simulink model "nonlinmodel"  (R2019b)
settings: Solver=VariableStepAuto  StartTime=0.0  StopTime=3000  RelTol=1e-3  EnableMultiTasking=on
values from neighbouring files (symbols this model uses):
  alpha = 0    [main.m]
  altitude = input('Enter the altitude for the simulation (ft)  :  ')    [main.m]
  Inertia = [9496,0,982 ... (first row only)    [main.m]
  mass = 636.94    [main.m]
  velocity = input('Enter the velocity for the simulation (ft/s):  ')    [main.m]
undefined symbols (not defined in the file or in its folder): U
libraries: aerolib6dof x4, simulink x4, aerolibobsolete x2, sharedutil x1
settings Model: Creator=Gray  LastModifiedBy=Administrator
settings DataIOCC: ReturnWorkspaceOutputs=off
settings OptimizationCC: LifeSpan=inf
settings DebuggingCC: SFUnexpectedBacktrackingDiag=warning  SFNoUnconditionalDefaultTransitionDiag=warning  ArithmeticOperatorsInVariantConditions=warning
settings SFSimCC: SimUseLocalCustomCode=off  CustomCodeUndefinedFunction=UseInterfaceOnly
settings RTWCC: RTWUseLocalCustomCode=off
settings CodeAppCC: StateflowObjectComments=on
settings GRTTargetCC: TargetLangStandard=C89/C90 (ANSI)  GeneratePreprocessorConditionals=Disable all
settings ConfigComp: CovMetricSettings=dw  CovHtmlReporting=on  CovSaveCumulativeToWorkspaceVar=on  CovSaveSingleToWorkspaceVar=on  CovExternalEMLEnable=off

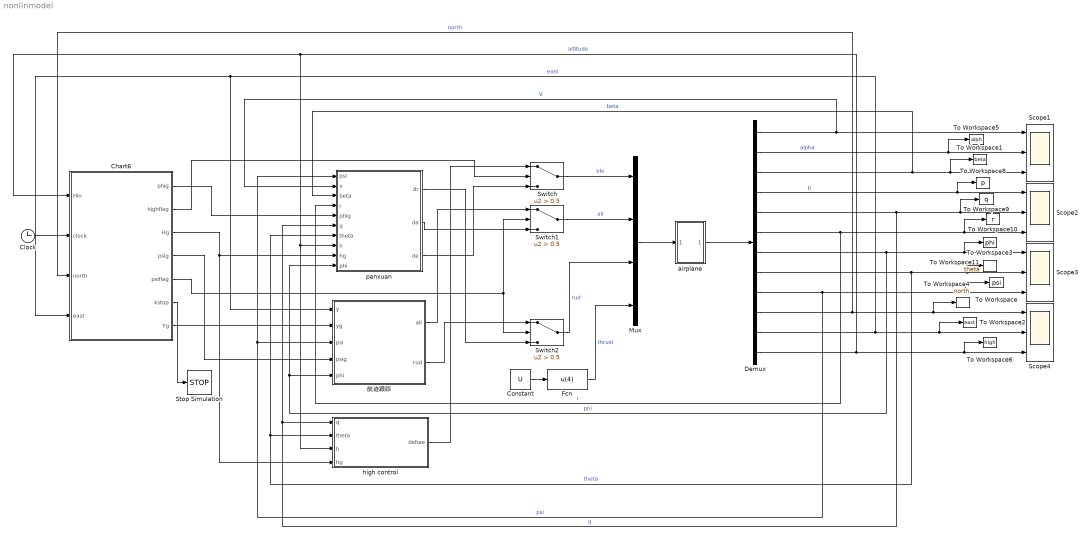
== system nonlinmodel ==
  Chart6 : Stateflow chart  TreatAsAtomicUnit=on
  Clock : Clock
  Constant : Constant  Value=U
  Demux : Demux  Outputs=12
  Fcn : Fcn  Expr=u(4)
  Mux : Mux
  Scope{1..4} (4 alike) : Scope  NumInputPorts=3
  Stop Simulation : Stop
  Switch : Switch  Criteria=u2 > Threshold  Threshold=0.5
  Switch1 : Switch  Criteria=u2 > Threshold  Threshold=0.5
  Switch2 : Switch  Criteria=u2 > Threshold  Threshold=0.5
  To Workspace : ToWorkspace  VariableName=psi  SaveFormat=Timeseries  SampleTime=-1
  To Workspace1 : ToWorkspace  VariableName=beta  SaveFormat=Timeseries  SampleTime=-1
  To Workspace10 : ToWorkspace  VariableName=r  SaveFormat=Timeseries  SampleTime=-1
  To Workspace11 : ToWorkspace  VariableName=theta  SaveFormat=Timeseries  SampleTime=-1
  To Workspace2 : ToWorkspace  VariableName=east  SampleTime=-1
  To Workspace3 : ToWorkspace  VariableName=phi  SaveFormat=Timeseries  SampleTime=-1
  To Workspace4 : ToWorkspace  VariableName=north  SampleTime=-1
  To Workspace5 : ToWorkspace  VariableName=alph  SaveFormat=Timeseries  SampleTime=-1
  To Workspace6 : ToWorkspace  VariableName=high  SampleTime=-1
      settings: Save2DSignal=2-D array (concatenate along first dimension)
  To Workspace8 : ToWorkspace  VariableName=p  SaveFormat=Timeseries  SampleTime=-1
  To Workspace9 : ToWorkspace  VariableName=q  SaveFormat=Timeseries  SampleTime=-1
  airplane : Subsystem
  high control : Subsystem
  panxuan : Subsystem
  航迹跟踪 : Subsystem
  wires:
  Demux/1 -> panxuan/2(v), Scope1/1  "V"
  Demux/2 -> To Workspace5/1, Scope1/2  "alpha"
  Demux/3 -> panxuan/3(beta), To Workspace1/1, Scope1/3  "beta"
  Demux/4 -> To Workspace8/1, Scope2/1  "p"
  Demux/5 -> panxuan/6(q), high control/1(q), To Workspace9/1, Scope2/2  "q"
  Demux/6 -> panxuan/4(r), To Workspace10/1, Scope2/3  "r"
  Demux/7 -> panxuan/10(phi), 航迹跟踪/5(phi), To Workspace3/1, Scope3/1  "phi"
  Demux/8 -> high control/2(theta), panxuan/7(theta), To Workspace11/1, Scope3/2  "theta"
  Demux/9 -> 航迹跟踪/3(psi), panxuan/1(psi), To Workspace/1, Scope3/3  "psi"
  Demux/10 -> Chart6/3(north), To Workspace4/1, Scope4/1  "north"
  Demux/11 -> Chart6/4(east), 航迹跟踪/1(y), To Workspace2/1, Scope4/2  "east"
  Demux/12 -> Chart6/1(Hin), high control/3(h), panxuan/8(h), To Workspace6/1, Scope4/3  "altitude"
  Fcn/1 -> Mux/4  "thrust"
  Chart6/1(phig) -> panxuan/5(phig)
  Chart6/3(Hg) -> high control/4(hg), panxuan/9(hg)
  Chart6/7(Yg) -> 航迹跟踪/2(yg)
  Chart6/4(psig) -> 航迹跟踪/4(psig)
  Switch/1 -> Mux/1  "ele"
  Switch1/1 -> Mux/2  "ail"
  Switch2/1 -> Mux/3  "rud"
  high control/1(deltae) -> Switch/1
  panxuan/3(de) -> Switch/3
  航迹跟踪/1(ail) -> Switch1/1
  panxuan/2(da) -> Switch1/3
  Chart6/2(highflag) -> Switch/2
  Chart6/5(psiflag) -> Switch2/2, Switch1/2
  Clock/1 -> Chart6/2(clock)
  Chart6/6(kstop) -> Stop Simulation/1
  航迹跟踪/2(rud) -> Switch2/1
  panxuan/1(dr) -> Switch2/3
  airplane/1(state) -> Demux/1
  Mux/1 -> airplane/1(In1)
  Constant/1 -> Fcn/1

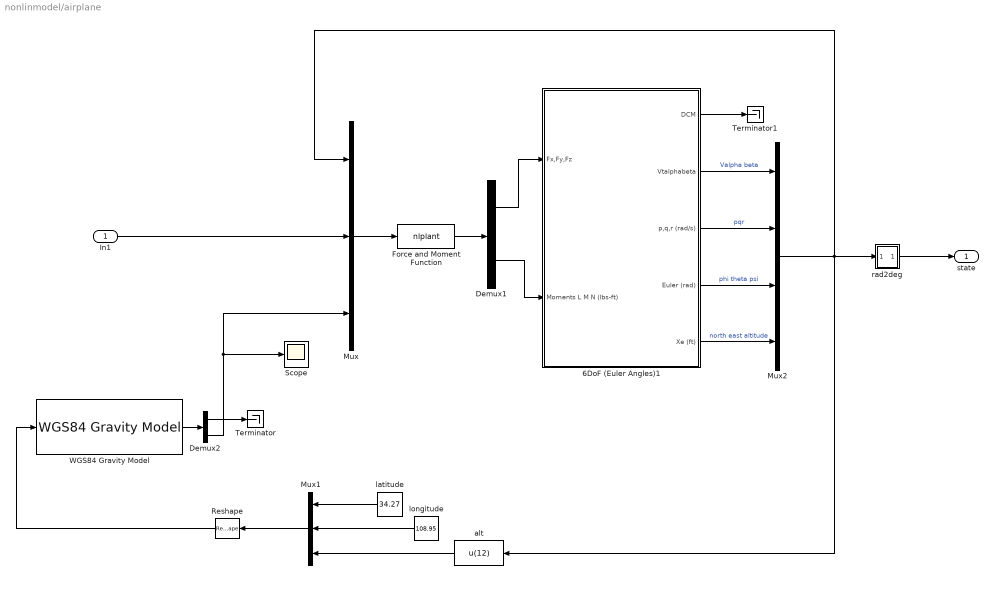
== system nonlinmodel/airplane ==
  In1 : Inport
  6DoF (Euler Angles)1 : Subsystem  RequirementInfo={} %GIDa_f78eee8a_25e5_4163_8dbf_11bc9aa697d0  AncestorBlock=aerolib6dof/6DoF (Euler Angles)  mask(6DoF (Euler Angles) EoM){xme_0=[0,0,altitude], Vmw_0=[velocity,alpha,0], eul_0=[0 0 0], pm_0=[0 0 0], mass=mass, Inertia=Inertia}
      mask prompts: xme_0 "Initial position in inertial axes [Xe,Ye,Ze] (ft):"; Vmw_0 "Vt  alpha  beta"; eul_0 "Initial Euler orientation [roll, pitch, yaw] (rad):"; pm_0 "Initial body rotation rates [p,q,r] (rad/s):"; mass "Mass (slugs):"; Inertia "Inertia matrix (slugs.ft^2):"
      mask help:
      | Integrate the six-degrees-of-freedom equations of motion using an Euler angle representation for the orientation of the body in space.
      |
      | Inputs are forces on the body in x-axis, y-axis, and z-axis; and moments on the body along x-axis, y-axis, and z-axis. Outputs are translational velocity in x-axis, y-axis, and z-axis in inertial coordinates; position in x-axis, y-axis, and z-axis in inertial coordinates; phi, theta, and psi; 3-by-3 direction cosine matrix; translational velocity in x-axis, y-axis, and z-axis in body coordinates; roll, pitch, and yaw rate; and roll, pitch, and yaw acceleration.
      mask Help: web(asbhelp('6dofeulerangles'));
      mask Display: disp('Euler\nAngles')
  Demux1 : Demux  Outputs=[3,3]
  Demux2 : Demux  Outputs=2
  Force and Moment Function : MATLABFcn  MATLABFcn=nlplant  OutputDimensions=6
  Mux : Mux  Inputs=[12,4,1]
  Mux1 : Mux  Inputs=3
  Mux2 : Mux
  Reshape : Reshape
  Scope : Scope
  Terminator : Terminator
  Terminator1 : Terminator
  "WGS84 Gravity Model " : aerolibobsolete/WGS84 Gravity Model   model=WGS84 Taylor Series  units=English  no_atmos=on  precessing=on  jd_loc=off  month=October  day=10  year=2004  no_centrifugal=on  action=Warning
      settings: SourceProductName=Aerospace Blockset  SourceProductBaseCode=AE
  alt : Fcn  Expr=u(12)
  latitude : Constant  Value=34.27
  longitude : Constant  Value=108.95
  rad2deg : Subsystem
  state : Outport
  wires:
  6DoF (Euler Angles)1/5(Xe (ft)) -> Mux2/4  "north east altitude"
  6DoF (Euler Angles)1/1(DCM) -> Terminator1/1
  rad2deg/1(Out1) -> state/1
  Force and Moment Function/1 -> Demux1/1
  latitude/1 -> Mux1/1
  Demux1/1 -> 6DoF (Euler Angles)1/1(Fx,Fy,Fz)
  Mux/1 -> Force and Moment Function/1
  In1/1 -> Mux/2
  Reshape/1 -> "WGS84 Gravity Model "/1
  alt/1 -> Mux1/3
  Demux1/2 -> 6DoF (Euler Angles)1/2(Moments L M N (lbs-ft))
  Demux2/2 -> Mux/3, Scope/1
  6DoF (Euler Angles)1/3(p,q,r (rad/s)) -> Mux2/2  "pqr"
  6DoF (Euler Angles)1/4(Euler (rad)) -> Mux2/3  "phi theta psi"
  Mux2/1 -> rad2deg/1(In1), alt/1, Mux/1
  longitude/1 -> Mux1/2
  Demux2/1 -> Terminator/1
  Mux1/1 -> Reshape/1
  "WGS84 Gravity Model "/1 -> Demux2/1
  6DoF (Euler Angles)1/2(Vtalphabeta) -> Mux2/1  "Valpha beta"

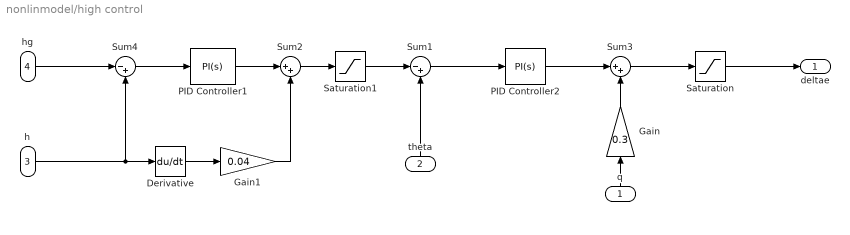
== system nonlinmodel/high control ==
  q : Inport
  theta : Inport  Port=2
  h : Inport  Port=3
  hg : Inport  Port=4
  Derivative : Derivative
  Gain : Gain  Gain=0.3
  Gain1 : Gain  Gain=0.04
  PID Controller1 : simulink/Continuous/PID Controller  Controller=PI  Form=Parallel  TimeDomain=Continuous-time  SampleTime=-1  IntegratorMethod=Forward Euler  FilterMethod=Forward Euler  ControllerParametersSource=internal  P=0.03  I=0.0002  D=0  UseFilter=on  N=100  TunerSelectOption=Transfer Function Based (PID Tuner App)  InitialConditionSource=internal  InitialConditionForIntegrator=0  InitialConditionForFilter=0  DifferentiatorICPrevScaledInput=0  ExternalReset=none  TrackingMode=off  Kt=1  LimitOutput=off  UpperSaturationLimit=inf  LowerSaturationLimit=-inf  LinearizeAsGain=on  AntiWindupMode=none  Kb=1  POutMin=[]  POutMax=[]  IOutMin=[]  IOutMax=[]  DOutMin=[]  DOutMax=[]  NOutMin=[]  NOutMax=[]  SumOutMin=[]  SumOutMax=[]  SaturationOutMin=[]  SaturationOutMax=[]  PParamMin=[]  PParamMax=[]  IParamMin=[]  IParamMax=[]  DParamMin=[]  DParamMax=[]  NParamMin=[]  NParamMax=[]  KbParamMin=[]  KbParamMax=[]  KtParamMin=[]  KtParamMax=[]  KbOutMin=[]  KbOutMax=[]  KtOutMin=[]  KtOutMax=[]  IntegratorOutMin=[]  IntegratorOutMax=[]  FilterOutMin=[]  FilterOutMax=[]  SumI1OutMin=[]  SumI1OutMax=[]  SumI2OutMin=[]  SumI2OutMax=[]  SumI3OutMin=[]  SumI3OutMax=[]  SumI4OutMin=[]  SumI4OutMax=[]  SumDOutMin=[]  SumDOutMax=[]  DifferentiatorOutMin=[]  DifferentiatorOutMax=[]  FilterDiffOutCoefMin=[]  FilterDiffOutCoefMax=[]  ReciprocalOutMin=[]  ReciprocalOutMax=[]  SumDenOutMin=[]  SumDenOutMax=[]  SumNumOutMin=[]  SumNumOutMax=[]  DivideOutMin=[]  DivideOutMax=[]  IntegratorContinuousStateAttributes=''  IntegratorStateMustResolveToSignalObject=off  IntegratorRTWStateStorageClass=Auto  FilterContinuousStateAttributes=''  FilterStateMustResolveToSignalObject=off  FilterRTWStateStorageClass=Auto  ParallelPVariant=InternalParameters  IdealPVariant=Disabled  IVariant=InternalParameters  DVariant=Disabled  IntegratorVariant=Continuous  SatVariant=Disabled  AWVariant=Passthrough  PCopyVariant=Disabled  TRVariant=Disabled  FdbkBlocksVariant=Forward  IdealPFdbkVariant=Disabled  SatFdbkVariant=Disabled  DerivativeFilterVariant=Disabled  NVariant=Disabled  NCopyVariant=Disabled_SignalSpec  FilterICVariant=Disabled  IntegratorICVariant=InternalICs  ExternalResetVariant=Disabled  TRSumVariant=Passthrough  SumFdbkVariant=Disabled  SumVariant=Sum_PI
  PID Controller2 : simulink/Continuous/PID Controller  Controller=PI  Form=Parallel  TimeDomain=Continuous-time  SampleTime=-1  IntegratorMethod=Forward Euler  FilterMethod=Forward Euler  ControllerParametersSource=internal  P=0.5  I=0  D=0  UseFilter=on  N=100  TunerSelectOption=Transfer Function Based (PID Tuner App)  InitialConditionSource=internal  InitialConditionForIntegrator=0  InitialConditionForFilter=0  DifferentiatorICPrevScaledInput=0  ExternalReset=none  TrackingMode=off  Kt=1  LimitOutput=off  UpperSaturationLimit=inf  LowerSaturationLimit=-inf  LinearizeAsGain=on  AntiWindupMode=none  Kb=1  POutMin=[]  POutMax=[]  IOutMin=[]  IOutMax=[]  DOutMin=[]  DOutMax=[]  NOutMin=[]  NOutMax=[]  SumOutMin=[]  SumOutMax=[]  SaturationOutMin=[]  SaturationOutMax=[]  PParamMin=[]  PParamMax=[]  IParamMin=[]  IParamMax=[]  DParamMin=[]  DParamMax=[]  NParamMin=[]  NParamMax=[]  KbParamMin=[]  KbParamMax=[]  KtParamMin=[]  KtParamMax=[]  KbOutMin=[]  KbOutMax=[]  KtOutMin=[]  KtOutMax=[]  IntegratorOutMin=[]  IntegratorOutMax=[]  FilterOutMin=[]  FilterOutMax=[]  SumI1OutMin=[]  SumI1OutMax=[]  SumI2OutMin=[]  SumI2OutMax=[]  SumI3OutMin=[]  SumI3OutMax=[]  SumI4OutMin=[]  SumI4OutMax=[]  SumDOutMin=[]  SumDOutMax=[]  DifferentiatorOutMin=[]  DifferentiatorOutMax=[]  FilterDiffOutCoefMin=[]  FilterDiffOutCoefMax=[]  ReciprocalOutMin=[]  ReciprocalOutMax=[]  SumDenOutMin=[]  SumDenOutMax=[]  SumNumOutMin=[]  SumNumOutMax=[]  DivideOutMin=[]  DivideOutMax=[]  IntegratorContinuousStateAttributes=''  IntegratorStateMustResolveToSignalObject=off  IntegratorRTWStateStorageClass=Auto  FilterContinuousStateAttributes=''  FilterStateMustResolveToSignalObject=off  FilterRTWStateStorageClass=Auto  ParallelPVariant=InternalParameters  IdealPVariant=Disabled  IVariant=InternalParameters  DVariant=Disabled  IntegratorVariant=Continuous  SatVariant=Disabled  AWVariant=Passthrough  PCopyVariant=Disabled  TRVariant=Disabled  FdbkBlocksVariant=Forward  IdealPFdbkVariant=Disabled  SatFdbkVariant=Disabled  DerivativeFilterVariant=Disabled  NVariant=Disabled  NCopyVariant=Disabled_SignalSpec  FilterICVariant=Disabled  IntegratorICVariant=InternalICs  ExternalResetVariant=Disabled  TRSumVariant=Passthrough  SumFdbkVariant=Disabled  SumVariant=Sum_PI
  Saturation : Saturate  UpperLimit=9  LowerLimit=-9
  Saturation1 : Saturate  UpperLimit=15  LowerLimit=-15
  Sum1 : Sum  Inputs=|-+
  Sum2 : Sum  Inputs=|++
  Sum3 : Sum  Inputs=|++
  Sum4 : Sum  Inputs=|-+
  deltae : Outport
  wires:
  hg/1 -> Sum4/1
  Sum4/1 -> PID Controller1/1
  PID Controller1/1 -> Sum2/1
  Sum1/1 -> PID Controller2/1
  PID Controller2/1 -> Sum3/1
  Sum3/1 -> Saturation/1
  h/1 -> Derivative/1, Sum4/2
  theta/1 -> Sum1/2
  Gain/1 -> Sum3/2
  q/1 -> Gain/1
  Saturation/1 -> deltae/1
  Saturation1/1 -> Sum1/1
  Sum2/1 -> Saturation1/1
  Derivative/1 -> Gain1/1
  Gain1/1 -> Sum2/2

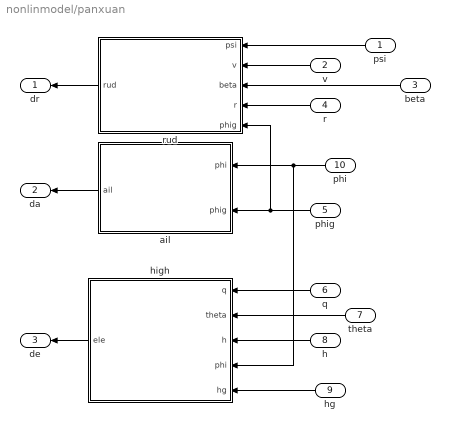
== system nonlinmodel/panxuan ==
  psi : Inport
  v : Inport  Port=2
  beta : Inport  Port=3
  r : Inport  Port=4
  phig : Inport  Port=5
  q : Inport  Port=6
  theta : Inport  Port=7
  h : Inport  Port=8
  hg : Inport  Port=9
  phi : Inport  Port=10
  ail : Subsystem
  "high " : Subsystem
  rud : Subsystem
  dr : Outport
  da : Outport  Port=2
  de : Outport  Port=3
  wires:
  psi/1 -> rud/1(psi)
  "high "/1(ele) -> de/1
  beta/1 -> rud/3(beta)
  r/1 -> rud/4(r)
  ail/1(ail) -> da/1
  v/1 -> rud/2(v)
  phig/1 -> rud/5(phig), ail/2(phig)
  theta/1 -> "high "/2(theta)
  q/1 -> "high "/1(q)
  h/1 -> "high "/3(h)
  hg/1 -> "high "/5(hg)
  rud/1(rud) -> dr/1
  phi/1 -> "high "/4(phi), ail/1(phi)

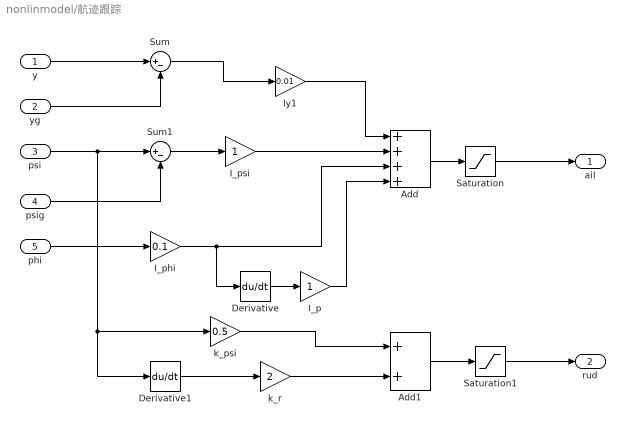
== system nonlinmodel/航迹跟踪 ==
  y : Inport
  yg : Inport  Port=2
  psi : Inport  Port=3
  psig : Inport  Port=4
  phi : Inport  Port=5
  Add : Sum  Inputs=++++
  Add1 : Sum
  Derivative : Derivative
  Derivative1 : Derivative
  I_p : Gain
  I_phi : Gain  Gain=0.1
  I_psi : Gain
  Iy1 : Gain  Gain=0.01
  Saturation : Saturate  UpperLimit=12  LowerLimit=-12
  Saturation1 : Saturate  UpperLimit=8  LowerLimit=-8
  Sum : Sum  Inputs=|+-
  Sum1 : Sum  Inputs=|+-
  k_psi : Gain  Gain=0.5
  k_r : Gain  Gain=2
  ail : Outport
  rud : Outport  Port=2
  wires:
  k_r/1 -> Add1/2
  k_psi/1 -> Add1/1
  Sum1/1 -> I_psi/1
  Add/1 -> Saturation/1
  Saturation/1 -> ail/1
  Add1/1 -> Saturation1/1
  Sum/1 -> Iy1/1
  Iy1/1 -> Add/1
  psi/1 -> Derivative1/1, k_psi/1, Sum1/1
  y/1 -> Sum/1
  psig/1 -> Sum1/2
  phi/1 -> I_phi/1
  I_phi/1 -> Derivative/1, Add/3
  Derivative/1 -> I_p/1
  Derivative1/1 -> k_r/1
  Saturation1/1 -> rud/1
  I_psi/1 -> Add/2
  I_p/1 -> Add/4
  yg/1 -> Sum/2

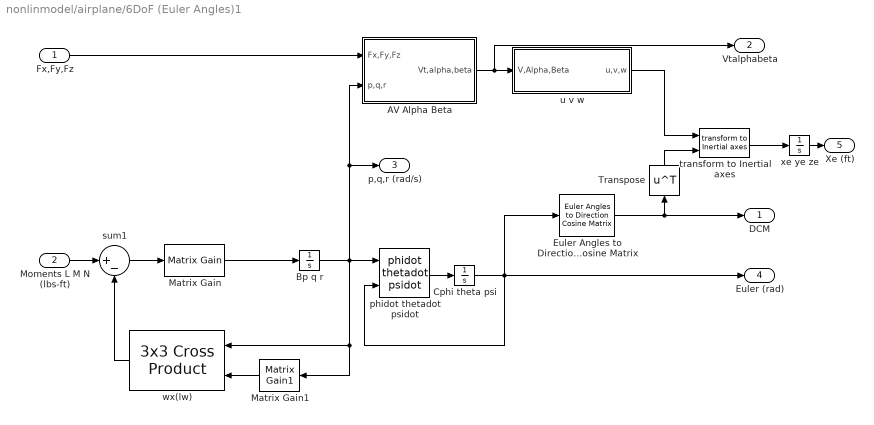
== system nonlinmodel/airplane/6DoF (Euler Angles)1 ==
  Fx,Fy,Fz : Inport  RequirementInfo={} %GIDa_47575797_6420_4b0e_a3a2_58bd686c73d1
  Moments L M N (lbs-ft) : Inport  RequirementInfo={} %GIDa_a1310ba6_e4bb_4a22_a342_2a9731745c55  Port=2
  AV Alpha Beta : Subsystem  RequirementInfo={} %GIDa_3bec4ccc_780c_4f29_8155_577fd785963f
  Bp q r : Integrator  RequirementInfo={} %GIDa_acd68407_7d65_4437_a75f_12a6524d518c  InitialCondition=pm_0
  Cphi theta psi : Integrator  RequirementInfo={} %GIDa_14df3cec_9b2c_44ff_9ee3_5db495ed21e4  InitialCondition=eul_0
  Euler Angles to Direction Cosine Matrix : aerolibobsolete/Euler Angles to  Direction Cosine Matrix
      settings: SourceProductName=Aerospace Blockset  SourceProductBaseCode=AE
  Matrix Gain : aerolib6dof/6DoF (Euler Angles)/Matrix Gain  K=inv(Inertia)
      settings: SourceProductName=Aerospace Blockset  SourceProductBaseCode=AE
  Matrix Gain1 : aerolib6dof/6DoF (Euler Angles)/Matrix Gain1  K=Inertia
      settings: SourceProductName=Aerospace Blockset  SourceProductBaseCode=AE
  Transpose : Math  RequirementInfo={} %GIDa_05e2ce72_03a0_43ff_82ff_9bf5926046c8  Operator=transpose  SaturateOnIntegerOverflow=on
  phidot thetadot psidot : aerolib6dof/6DoF (Euler Angles)/phidot thetadot psidot  SystemSampleTime=-1  Latency=0  AutoFrameSizeCalculation=off
      settings: SourceProductName=Aerospace Blockset  SourceProductBaseCode=AE
  sum1 : Sum  RequirementInfo={} %GIDa_32be784a_f452_4b23_b55c_981dfbd798a6  Inputs=|+-  SaturateOnIntegerOverflow=on  InputSameDT=on  OutDataTypeStr=Inherit: Same as first input
  "transform to Inertial axes " : aerolib6dof/6DoF (Euler Angles)/transform to Inertial axes   SystemSampleTime=-1  Latency=0  AutoFrameSizeCalculation=off
      settings: SourceProductName=Aerospace Blockset  SourceProductBaseCode=AE
  u v w : Subsystem  RequirementInfo={} %GIDa_bf3c1f97_35ea_453e_a36d_366a8121257e
  wx(lw) : sharedutil/3x3 Cross Product  aMode=aMode
      settings: SourceProductBaseCode=AE
  xe ye ze : Integrator  RequirementInfo={} %GIDa_cfcfa943_adf2_4818_a2ff_e6c6db1ce85e  InitialCondition=xme_0
  DCM : Outport  RequirementInfo={} %GIDa_e636d6ae_e403_4b09_a804_1aa986cdae3b
  Vtalphabeta : Outport  RequirementInfo={} %GIDa_aa55a071_a531_47c1_a623_ce86d5a78c20  Port=2
  p,q,r (rad/s) : Outport  RequirementInfo={} %GIDa_fd949a73_e74c_4d0d_912e_86edec8a02c0  Port=3
  Euler (rad) : Outport  RequirementInfo={} %GIDa_0d674778_96dd_4688_9946_da01fc5c90ef  Port=4
  Xe (ft) : Outport  RequirementInfo={} %GIDa_d3340636_7588_4a71_8e89_73856e7a4ca7  Port=5
  wires:
  Transpose/1 -> "transform to Inertial axes "/2
  Euler Angles to Direction Cosine Matrix/1 -> Transpose/1, DCM/1
  Matrix Gain/1 -> Bp q r/1
  wx(lw)/1 -> sum1/2
  Matrix Gain1/1 -> wx(lw)/2
  Moments L M N (lbs-ft)/1 -> sum1/1
  sum1/1 -> Matrix Gain/1
  Bp q r/1 -> Matrix Gain1/1, wx(lw)/1, phidot thetadot psidot/1, p,q,r (rad/s)/1, AV Alpha Beta/2(p,q,r)
  "transform to Inertial axes "/1 -> xe ye ze/1
  xe ye ze/1 -> Xe (ft)/1
  u v w/1(u,v,w) -> "transform to Inertial axes "/1
  Cphi theta psi/1 -> phidot thetadot psidot/2, Euler Angles to Direction Cosine Matrix/1, Euler (rad)/1
  phidot thetadot psidot/1 -> Cphi theta psi/1
  AV Alpha Beta/1(Vt,alpha,beta) -> Vtalphabeta/1, u v w/1(V,Alpha,Beta)
  Fx,Fy,Fz/1 -> AV Alpha Beta/1(Fx,Fy,Fz)

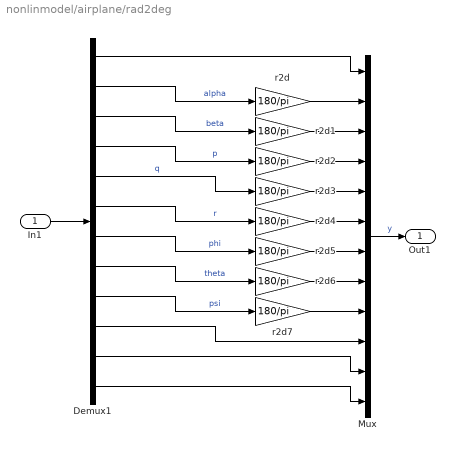
== system nonlinmodel/airplane/rad2deg ==
  In1 : Inport
  Demux1 : Demux  Outputs=12
  Mux : Mux  Inputs=12
  r2d{,1..7} (8 alike) : Gain  Gain=180/pi  SaturateOnIntegerOverflow=on  OutDataTypeStr=Inherit: Same as input  ParamDataTypeStr=Inherit: Same as input
  Out1 : Outport
  wires:
  In1/1 -> Demux1/1
  r2d2/1 -> Mux/4
  r2d1/1 -> Mux/3
  r2d/1 -> Mux/2
  Mux/1 -> Out1/1  "y"
  Demux1/1 -> Mux/1
  Demux1/2 -> r2d/1  "alpha"
  Demux1/3 -> r2d1/1  "beta"
  Demux1/4 -> r2d2/1  "p"
  Demux1/5 -> r2d3/1  "q"
  r2d3/1 -> Mux/5
  r2d4/1 -> Mux/6
  r2d5/1 -> Mux/7
  r2d6/1 -> Mux/8
  r2d7/1 -> Mux/9
  Demux1/6 -> r2d4/1  "r"
  Demux1/7 -> r2d5/1  "phi"
  Demux1/8 -> r2d6/1  "theta"
  Demux1/9 -> r2d7/1  "psi"
  Demux1/10 -> Mux/10
  Demux1/11 -> Mux/11
  Demux1/12 -> Mux/12

== system nonlinmodel/panxuan/ail ==
  phi : Inport
  phig : Inport  Port=2
  Add : Sum  Inputs=-+
  Add1 : Sum  Inputs=+++
  Derivative : Derivative
  Gain1 : Gain  Gain=0.4
  Gain2 : Gain
  Gain3 : Gain
  Integrator : Integrator
  Saturation : Saturate  UpperLimit=12  LowerLimit=-12
  ail : Outport
  wires:
  phi/1 -> Derivative/1, Add/2, Gain2/1
  Add1/1 -> Saturation/1
  Add/1 -> Integrator/1
  Integrator/1 -> Gain1/1
  Saturation/1 -> ail/1
  phig/1 -> Add/1
  Derivative/1 -> Gain3/1
  Gain2/1 -> Add1/2
  Gain3/1 -> Add1/3
  Gain1/1 -> Add1/1

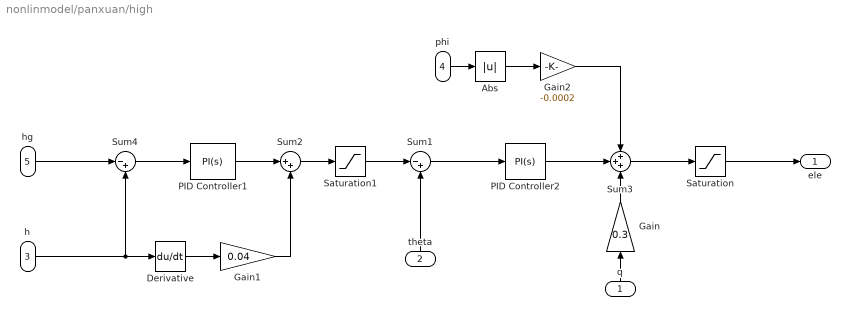
== system nonlinmodel/panxuan/high  ==
  q : Inport
  theta : Inport  Port=2
  h : Inport  Port=3
  phi : Inport  Port=4
  hg : Inport  Port=5
  Abs : Abs
  Derivative : Derivative
  Gain : Gain  Gain=0.3
  Gain1 : Gain  Gain=0.04
  Gain2 : Gain  Gain=-0.0002
  PID Controller1 : simulink/Continuous/PID Controller  Controller=PI  Form=Parallel  TimeDomain=Continuous-time  SampleTime=-1  IntegratorMethod=Forward Euler  FilterMethod=Forward Euler  ControllerParametersSource=internal  P=0.03  I=0.0002  D=0  UseFilter=on  N=100  TunerSelectOption=Transfer Function Based (PID Tuner App)  InitialConditionSource=internal  InitialConditionForIntegrator=0  InitialConditionForFilter=0  DifferentiatorICPrevScaledInput=0  ExternalReset=none  TrackingMode=off  Kt=1  LimitOutput=off  UpperSaturationLimit=inf  LowerSaturationLimit=-inf  LinearizeAsGain=on  AntiWindupMode=none  Kb=1  POutMin=[]  POutMax=[]  IOutMin=[]  IOutMax=[]  DOutMin=[]  DOutMax=[]  NOutMin=[]  NOutMax=[]  SumOutMin=[]  SumOutMax=[]  SaturationOutMin=[]  SaturationOutMax=[]  PParamMin=[]  PParamMax=[]  IParamMin=[]  IParamMax=[]  DParamMin=[]  DParamMax=[]  NParamMin=[]  NParamMax=[]  KbParamMin=[]  KbParamMax=[]  KtParamMin=[]  KtParamMax=[]  KbOutMin=[]  KbOutMax=[]  KtOutMin=[]  KtOutMax=[]  IntegratorOutMin=[]  IntegratorOutMax=[]  FilterOutMin=[]  FilterOutMax=[]  SumI1OutMin=[]  SumI1OutMax=[]  SumI2OutMin=[]  SumI2OutMax=[]  SumI3OutMin=[]  SumI3OutMax=[]  SumI4OutMin=[]  SumI4OutMax=[]  SumDOutMin=[]  SumDOutMax=[]  DifferentiatorOutMin=[]  DifferentiatorOutMax=[]  FilterDiffOutCoefMin=[]  FilterDiffOutCoefMax=[]  ReciprocalOutMin=[]  ReciprocalOutMax=[]  SumDenOutMin=[]  SumDenOutMax=[]  SumNumOutMin=[]  SumNumOutMax=[]  DivideOutMin=[]  DivideOutMax=[]  IntegratorContinuousStateAttributes=''  IntegratorStateMustResolveToSignalObject=off  IntegratorRTWStateStorageClass=Auto  FilterContinuousStateAttributes=''  FilterStateMustResolveToSignalObject=off  FilterRTWStateStorageClass=Auto  ParallelPVariant=InternalParameters  IdealPVariant=Disabled  IVariant=InternalParameters  DVariant=Disabled  IntegratorVariant=Continuous  SatVariant=Disabled  AWVariant=Passthrough  PCopyVariant=Disabled  TRVariant=Disabled  FdbkBlocksVariant=Forward  IdealPFdbkVariant=Disabled  SatFdbkVariant=Disabled  DerivativeFilterVariant=Disabled  NVariant=Disabled  NCopyVariant=Disabled_SignalSpec  FilterICVariant=Disabled  IntegratorICVariant=InternalICs  ExternalResetVariant=Disabled  TRSumVariant=Passthrough  SumFdbkVariant=Disabled  SumVariant=Sum_PI
  PID Controller2 : simulink/Continuous/PID Controller  Controller=PI  Form=Parallel  TimeDomain=Continuous-time  SampleTime=-1  IntegratorMethod=Forward Euler  FilterMethod=Forward Euler  ControllerParametersSource=internal  P=0.5  I=0  D=0  UseFilter=on  N=100  TunerSelectOption=Transfer Function Based (PID Tuner App)  InitialConditionSource=internal  InitialConditionForIntegrator=0  InitialConditionForFilter=0  DifferentiatorICPrevScaledInput=0  ExternalReset=none  TrackingMode=off  Kt=1  LimitOutput=off  UpperSaturationLimit=inf  LowerSaturationLimit=-inf  LinearizeAsGain=on  AntiWindupMode=none  Kb=1  POutMin=[]  POutMax=[]  IOutMin=[]  IOutMax=[]  DOutMin=[]  DOutMax=[]  NOutMin=[]  NOutMax=[]  SumOutMin=[]  SumOutMax=[]  SaturationOutMin=[]  SaturationOutMax=[]  PParamMin=[]  PParamMax=[]  IParamMin=[]  IParamMax=[]  DParamMin=[]  DParamMax=[]  NParamMin=[]  NParamMax=[]  KbParamMin=[]  KbParamMax=[]  KtParamMin=[]  KtParamMax=[]  KbOutMin=[]  KbOutMax=[]  KtOutMin=[]  KtOutMax=[]  IntegratorOutMin=[]  IntegratorOutMax=[]  FilterOutMin=[]  FilterOutMax=[]  SumI1OutMin=[]  SumI1OutMax=[]  SumI2OutMin=[]  SumI2OutMax=[]  SumI3OutMin=[]  SumI3OutMax=[]  SumI4OutMin=[]  SumI4OutMax=[]  SumDOutMin=[]  SumDOutMax=[]  DifferentiatorOutMin=[]  DifferentiatorOutMax=[]  FilterDiffOutCoefMin=[]  FilterDiffOutCoefMax=[]  ReciprocalOutMin=[]  ReciprocalOutMax=[]  SumDenOutMin=[]  SumDenOutMax=[]  SumNumOutMin=[]  SumNumOutMax=[]  DivideOutMin=[]  DivideOutMax=[]  IntegratorContinuousStateAttributes=''  IntegratorStateMustResolveToSignalObject=off  IntegratorRTWStateStorageClass=Auto  FilterContinuousStateAttributes=''  FilterStateMustResolveToSignalObject=off  FilterRTWStateStorageClass=Auto  ParallelPVariant=InternalParameters  IdealPVariant=Disabled  IVariant=InternalParameters  DVariant=Disabled  IntegratorVariant=Continuous  SatVariant=Disabled  AWVariant=Passthrough  PCopyVariant=Disabled  TRVariant=Disabled  FdbkBlocksVariant=Forward  IdealPFdbkVariant=Disabled  SatFdbkVariant=Disabled  DerivativeFilterVariant=Disabled  NVariant=Disabled  NCopyVariant=Disabled_SignalSpec  FilterICVariant=Disabled  IntegratorICVariant=InternalICs  ExternalResetVariant=Disabled  TRSumVariant=Passthrough  SumFdbkVariant=Disabled  SumVariant=Sum_PI
  Saturation : Saturate  UpperLimit=9  LowerLimit=-9
  Saturation1 : Saturate  UpperLimit=15  LowerLimit=-15
  Sum1 : Sum  Inputs=|-+
  Sum2 : Sum  Inputs=|++
  Sum3 : Sum  Inputs=+++
  Sum4 : Sum  Inputs=|-+
  ele : Outport
  wires:
  hg/1 -> Sum4/1
  Sum4/1 -> PID Controller1/1
  PID Controller1/1 -> Sum2/1
  Sum1/1 -> PID Controller2/1
  Sum3/1 -> Saturation/1
  h/1 -> Derivative/1, Sum4/2
  theta/1 -> Sum1/2
  q/1 -> Gain/1
  Saturation/1 -> ele/1
  Saturation1/1 -> Sum1/1
  Sum2/1 -> Saturation1/1
  Derivative/1 -> Gain1/1
  Gain1/1 -> Sum2/2
  PID Controller2/1 -> Sum3/2
  Gain/1 -> Sum3/3
  phi/1 -> Abs/1
  Abs/1 -> Gain2/1
  Gain2/1 -> Sum3/1

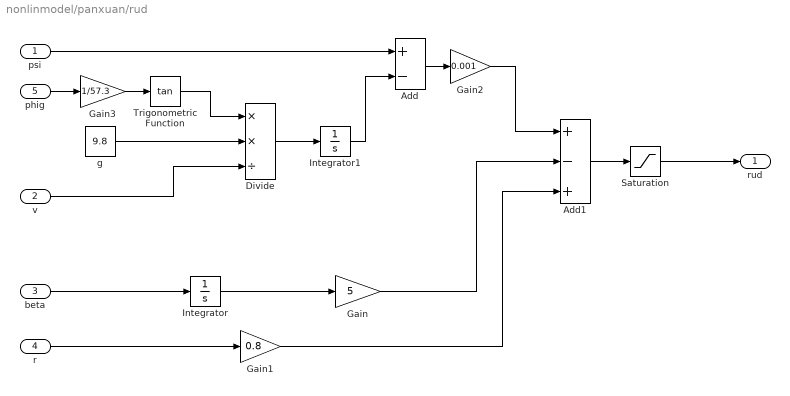
== system nonlinmodel/panxuan/rud ==
  psi : Inport
  v : Inport  Port=2
  beta : Inport  Port=3
  r : Inport  Port=4
  phig : Inport  Port=5
  Add : Sum  Inputs=+-
  Add1 : Sum  Inputs=+-+
  Divide : Product  Inputs=**/
  Gain : Gain  Gain=5
  Gain1 : Gain  Gain=0.8
  Gain2 : Gain  Gain=0.001
  Gain3 : Gain  Gain=1/57.3
  Integrator : Integrator
  Integrator1 : Integrator
  Saturation : Saturate  UpperLimit=8  LowerLimit=-8
  Trigonometric Function : Trigonometry  Operator=tan
  g : Constant  Value=9.8
  rud : Outport
  wires:
  Saturation/1 -> rud/1
  Add1/1 -> Saturation/1
  Trigonometric Function/1 -> Divide/1
  g/1 -> Divide/2
  psi/1 -> Add/1
  Add/1 -> Gain2/1
  r/1 -> Gain1/1
  Divide/1 -> Integrator1/1
  Integrator1/1 -> Add/2
  v/1 -> Divide/3
  Gain1/1 -> Add1/3
  Integrator/1 -> Gain/1
  beta/1 -> Integrator/1
  Gain2/1 -> Add1/1
  Gain/1 -> Add1/2
  phig/1 -> Gain3/1
  Gain3/1 -> Trigonometric Function/1

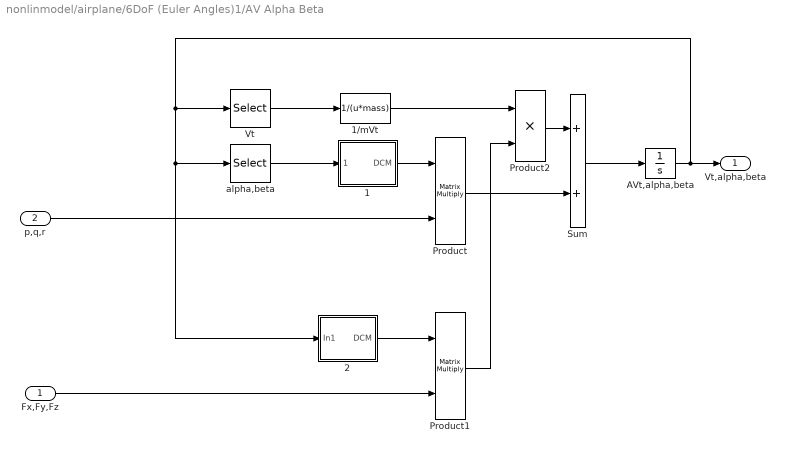
== system nonlinmodel/airplane/6DoF (Euler Angles)1/AV Alpha Beta ==
  Fx,Fy,Fz : Inport  RequirementInfo={} %GIDa_3a0cf2a3_c1ed_4a73_94fd_889fed1d9b56
  p,q,r : Inport  RequirementInfo={} %GIDa_a5f9e550_3eab_4ac3_94b5_06fdd9a422da  Port=2
  1 : Subsystem  RequirementInfo={} %GIDa_c99e5cc3_cc96_42d4_9ef2_1efd010a1b78  AncestorBlock="aerolibtransform/Euler Angles to  Direction Cosine Matrix"  mask(Euler2DCM){}
      mask help: Determine the 3-by-3 direction cosine matrix (DCM) from an Euler orientation (roll, pitch, yaw). The output DCM transforms vectors from inertial axes to body axes.
      mask Help: web(asbhelp('euleranglestodirectioncosinematrix'));
      mask Display: disp('Eul2DCM')
  1/mVt : Fcn  RequirementInfo={} %GIDa_624a88a3_87d0_4b9d_baa6_8a4cfcde3bec  Expr=1/(u*mass)
  2 : Subsystem  RequirementInfo={} %GIDa_e3eb13bd_00a3_4e12_afed_b34375ccdab9  AncestorBlock="aerolibtransform/Euler Angles to  Direction Cosine Matrix"  mask(Euler2DCM){}
      mask help: Determine the 3-by-3 direction cosine matrix (DCM) from an Euler orientation (roll, pitch, yaw). The output DCM transforms vectors from inertial axes to body axes.
      mask Help: web(asbhelp('euleranglestodirectioncosinematrix'));
      mask Display: disp('Eul2DCM')
  AVt,alpha,beta : Integrator  RequirementInfo={} %GIDa_5872e78a_3bc5_4f03_9b8b_91f33d6f31ba  InitialCondition=Vmw_0
  Product : Product  RequirementInfo={} %GIDa_2274bb0d_f78c_488a_822a_45d167d88f93  Multiplication=Matrix(*)  SaturateOnIntegerOverflow=on  OutDataTypeStr=Inherit: Same as first input
  Product1 : Product  RequirementInfo={} %GIDa_0f8d436f_1e01_4328_91a6_d2bc540051ee  Multiplication=Matrix(*)  SaturateOnIntegerOverflow=on  OutDataTypeStr=Inherit: Same as first input
  Product2 : Product  RequirementInfo={} %GIDa_e5f757ea_6d25_4229_bd39_4205d2ac714e  SaturateOnIntegerOverflow=on  OutDataTypeStr=Inherit: Same as first input
  Sum : Sum  RequirementInfo={} %GIDa_dca47486_89f6_482a_88b1_b8e711c95790  SaturateOnIntegerOverflow=on
  Vt : Selector  RequirementInfo={} %GIDa_5895aaee_ce00_487e_a691_99d90d7f70b9  InputPortWidth=3  IndexOptions=Index vector (dialog)  Indices=[1]  OutputSizes=1
  alpha,beta : Selector  RequirementInfo={} %GIDa_af6a7055_0671_43e6_ae58_ce8d0b3d3dfc  InputPortWidth=3  IndexOptions=Index vector (dialog)  Indices=[2 3]  OutputSizes=1
  Vt,alpha,beta : Outport  RequirementInfo={} %GIDa_cdaa0784_0bf0_4f30_8d27_66f252016894
  wires:
  1/1(DCM) -> Product/1
  p,q,r/1 -> Product/2
  2/1(DCM) -> Product1/1
  alpha,beta/1 -> 1/1(aeodata)
  Fx,Fy,Fz/1 -> Product1/2
  Vt/1 -> 1/mVt/1
  Product1/1 -> Product2/2
  1/mVt/1 -> Product2/1
  Product2/1 -> Sum/1
  Product/1 -> Sum/2
  Sum/1 -> AVt,alpha,beta/1
  AVt,alpha,beta/1 -> Vt,alpha,beta/1, Vt/1, 2/1(In1), alpha,beta/1

== system nonlinmodel/airplane/6DoF (Euler Angles)1/u v w ==
  V,Alpha,Beta : Inport  RequirementInfo={} %GIDa_c914807c_377c_4805_904c_b9dd6b416fbe
  11 : Fcn  RequirementInfo={} %GIDa_d585e0af_bb62_4f73_bfd9_c6723cca6caa  Expr=u(3)*u(4)*u(5)
  21 : Fcn  RequirementInfo={} %GIDa_43b00716_1676_4525_a1fa_24f1ca32aa06  Expr=u(2)*u(5)
  31 : Fcn  RequirementInfo={} %GIDa_18e180b3_585b_4d34_a8cd_b377e391badc  Expr=u(1)*u(4)*u(5)
  Demux : Demux  RequirementInfo={} %GIDa_6872fdb6_9740_423d_ad70_4060b7917c22  Outputs=[1,2]
  Mux : Mux  RequirementInfo={} %GIDa_6855cb8d_5fe5_474e_adbb_e3179ac4eebe  Inputs=3
  Mux1 : Mux  RequirementInfo={} %GIDa_6d5c0bc9_39df_4fb1_b18d_a12a1f469acd  Inputs=3
  cos(alpha,beta) : Trigonometry  RequirementInfo={} %GIDa_de370d12_4345_49dc_94a0_85fda68f9318  Operator=cos
  sin(alpha,beta) : Trigonometry  RequirementInfo={} %GIDa_6f775f89_370c_4c24_bd51_5746d9ad32c3
  u,v,w : Outport  RequirementInfo={} %GIDa_faedc8a5_0e93_4459_a6c9_fe783164ef2e
  wires:
  V,Alpha,Beta/1 -> Demux/1
  Mux1/1 -> u,v,w/1
  sin(alpha,beta)/1 -> Mux/1
  cos(alpha,beta)/1 -> Mux/2
  Mux/1 -> 11/1, 21/1, 31/1
  Demux/1 -> Mux/3
  11/1 -> Mux1/1
  21/1 -> Mux1/2
  31/1 -> Mux1/3
  Demux/2 -> sin(alpha,beta)/1, cos(alpha,beta)/1

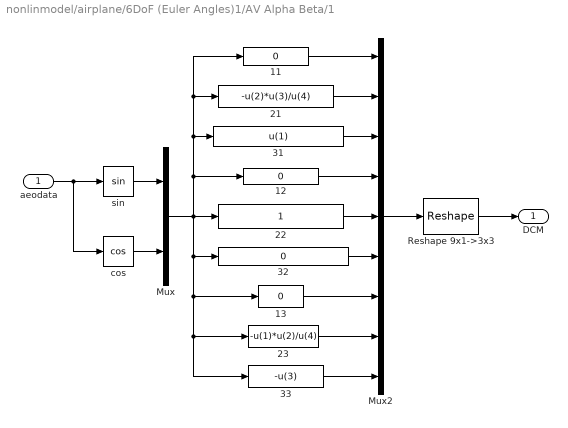
== system nonlinmodel/airplane/6DoF (Euler Angles)1/AV Alpha Beta/1 ==
  aeodata : Inport  RequirementInfo={} %GIDa_26334d88_e482_484f_b2e7_c9fa6d526c27
  11 : Fcn  RequirementInfo={} %GIDa_3b64c8f2_ebc0_426a_a0b0_8d1b09163b48  Expr=0
  12 : Fcn  RequirementInfo={} %GIDa_62435e47_a87c_4dcd_b50e_177845bffaf0  Expr=0
  13 : Fcn  RequirementInfo={} %GIDa_1b5cde54_80f2_453f_8970_fe6aea009974  Expr=0
  21 : Fcn  RequirementInfo={} %GIDa_bd0fbc7c_0fa4_407c_a960_55cbadc205e2  Expr=-u(2)*u(3)/u(4)
  22 : Fcn  RequirementInfo={} %GIDa_b9d67027_81e2_441a_be1e_54c25a531490  Expr=1
  23 : Fcn  RequirementInfo={} %GIDa_5b34ddd2_f10b_46f3_a37d_d3db88c149ce  Expr=-u(1)*u(2)/u(4)
  31 : Fcn  RequirementInfo={} %GIDa_c0edd0fb_54b7_4d9b_996f_cd482e49dd82  Expr=u(1)
  32 : Fcn  RequirementInfo={} %GIDa_f063a6a6_3071_4678_ae87_0d85f85bf8e7  Expr=0
  33 : Fcn  RequirementInfo={} %GIDa_8e91e91c_cea0_4225_b517_e6ef505d02c9  Expr=-u(3)
  Mux : Mux  RequirementInfo={} %GIDa_533c009e_0b36_44d6_89a0_d85a9332b8c0  Inputs=2
  Mux2 : Mux  RequirementInfo={} %GIDa_01f06579_276f_4188_a891_ef4ef8fa48ef  Inputs=9
  Reshape 9x1->3x3 : Reshape  RequirementInfo={} %GIDa_f87fc956_d370_46d1_9810_e7adad4a2eed  OutputDimensionality=Customize  OutputDimensions=[3,3]
  cos : Trigonometry  RequirementInfo={} %GIDa_e724210f_fb03_4dde_aece_76312382e649  Operator=cos
  sin : Trigonometry  RequirementInfo={} %GIDa_e4915e86_d752_4f6e_aa35_24073a1246c8
  DCM : Outport  RequirementInfo={} %GIDa_0ccdfa7e_6a60_431c_9fd0_97638da1abe3  InitialOutput=0
  wires:
  33/1 -> Mux2/9
  23/1 -> Mux2/8
  13/1 -> Mux2/7
  32/1 -> Mux2/6
  22/1 -> Mux2/5
  12/1 -> Mux2/4
  31/1 -> Mux2/3
  21/1 -> Mux2/2
  11/1 -> Mux2/1
  Mux2/1 -> Reshape 9x1->3x3/1
  Reshape 9x1->3x3/1 -> DCM/1
  sin/1 -> Mux/1
  cos/1 -> Mux/2
  aeodata/1 -> sin/1, cos/1
  Mux/1 -> 22/1, 11/1, 21/1, 31/1, 12/1, 32/1, 13/1, 23/1, 33/1

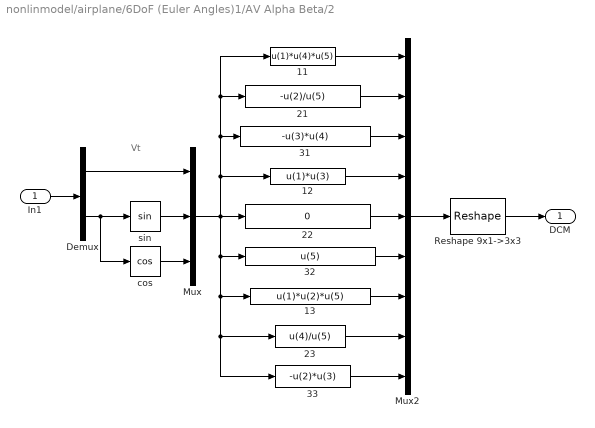
== system nonlinmodel/airplane/6DoF (Euler Angles)1/AV Alpha Beta/2 ==
  note: Vt
  In1 : Inport  RequirementInfo={} %GIDa_36cbbc4a_b3c2_4845_bb6d_f0c8800e9bb0
  11 : Fcn  RequirementInfo={} %GIDa_a7e6f812_ab30_41d5_89de_99289fb1c9f0  Expr=u(1)*u(4)*u(5)
  12 : Fcn  RequirementInfo={} %GIDa_f8d10927_5a8d_4480_869c_a5e5f8b64f32  Expr=u(1)*u(3)
  13 : Fcn  RequirementInfo={} %GIDa_38a6d479_343a_4a9c_8249_b658f7d736e2  Expr=u(1)*u(2)*u(5)
  21 : Fcn  RequirementInfo={} %GIDa_03ff6ab3_928c_409e_b16c_df97aa4c986c  Expr=-u(2)/u(5)
  22 : Fcn  RequirementInfo={} %GIDa_bb32bd65_5533_4481_915c_09e89aa98e1f  Expr=0
  23 : Fcn  RequirementInfo={} %GIDa_16ad9f63_ee2e_4756_a565_07aecda4ca7d  Expr=u(4)/u(5)
  31 : Fcn  RequirementInfo={} %GIDa_5e578829_25d6_4bb1_9e28_75bfeeb305da  Expr=-u(3)*u(4)
  32 : Fcn  RequirementInfo={} %GIDa_e8186994_ab00_4082_bac3_5117986a1dd8  Expr=u(5)
  33 : Fcn  RequirementInfo={} %GIDa_857ef62e_78e0_4aa9_89ea_123a28525025  Expr=-u(2)*u(3)
  Demux : Demux  RequirementInfo={} %GIDa_ab63bb57_9ca0_4c67_b452_c12ab2673a7c  Outputs=[1 2]
  Mux : Mux  RequirementInfo={} %GIDa_fa29df0f_2cee_4dab_bf98_983935ed2095  Inputs=[1 2 2]
  Mux2 : Mux  RequirementInfo={} %GIDa_e567c283_4285_49ee_a5b5_4d615cd21c9e  Inputs=9
  Reshape 9x1->3x3 : Reshape  RequirementInfo={} %GIDa_b468087c_a202_4f9e_9d80_8b39de33c9b5  OutputDimensionality=Customize  OutputDimensions=[3,3]
  cos : Trigonometry  RequirementInfo={} %GIDa_5526c739_d71a_4e6c_a0dd_da01aca85f40  Operator=cos
  sin : Trigonometry  RequirementInfo={} %GIDa_aef9b91e_0ef8_4b58_a89f_3d0eee804f88
  DCM : Outport  RequirementInfo={} %GIDa_e04188f2_f8ca_4551_b78a_ff264537c622  InitialOutput=0
  wires:
  Mux/1 -> 33/1, 23/1, 13/1, 32/1, 12/1, 31/1, 21/1, 11/1, 22/1
  Demux/2 -> cos/1, sin/1
  Reshape 9x1->3x3/1 -> DCM/1
  Mux2/1 -> Reshape 9x1->3x3/1
  11/1 -> Mux2/1
  21/1 -> Mux2/2
  31/1 -> Mux2/3
  12/1 -> Mux2/4
  22/1 -> Mux2/5
  32/1 -> Mux2/6
  13/1 -> Mux2/7
  23/1 -> Mux2/8
  33/1 -> Mux2/9
  sin/1 -> Mux/2
  cos/1 -> Mux/3
  Demux/1 -> Mux/1
  In1/1 -> Demux/1

== stateflow chart nonlinmodel/Chart6 ==
  state panxuan
    entry:highflag=0;
    Hg=22000;psig=0;psiflag=0;
    Yg=100;phig=10;
    exit:tt3=clock;
  state pingfei1
    entry:highflag=1;
    Hg=21800;psig=0;psiflag=1;
    Yg=0;phig=0;
  state xiahua
    entry:highflag=1;
    Hg=22000;psig=0;psiflag=1;
    Yg=0;phig=0;
    exit: tt2=clock;
  state pingfei
    entry:highflag=1;
    Hg=22000;psig=0;psiflag=1;
    Yg=0;phig=0;
  state pasheng
    entry:highflag=1;
    Hg=21800;psig=0;psiflag=1;
    Yg=0;phig=0;
    exit: tt1=clock;
  state pingfei4
    entry:highflag=1;
    Hg=22000;psig=0;psiflag=1;
    Yg=100;phig=0;
  state stop
    entry:kstop=1;
  state pingfei3
    entry:highflag=1;
    Hg=22000;psig=0;psiflag=1;
    Yg=0;phig=0;
  state cepian
    entry:highflag=1;
    Hg=22000;psig=0;psiflag=1;
    Yg=100;phig=0;
  (default) -> pingfei
  pingfei1 -> xiahua : [clock>tt1+40]
  panxuan -> stop : [clock>tt3+1500]
  pingfei4 -> panxuan : [sqrt((north-500000)^2+(east-Yg)^2)<100]
  pasheng -> pingfei1 : [(Hin>=21795)&&(Hin<=21805)]
  xiahua -> pingfei3 : [(Hin>=21995)&&(Hin<=22005)]
  pingfei -> pasheng : [clock>20]
  cepian -> pingfei4 : [(east>95)&&(east<105)]
  pingfei3 -> cepian : [clock>tt2+20]
  data: Hin input double; phig output double; highflag output double; clock input double; Hg output double; psig output double; psiflag output double; kstop output double; north input double; east input double; Yg output double; tt1 local double; tt2 local double; tt3 local double
